simulink model "PI"  (R2015a)
settings: Solver=ode45  StartTime=0.0  StopTime=300  RelTol=1e-3
libraries: fuzblock x1
settings Model: Creator=Q  LastModifiedBy=Q

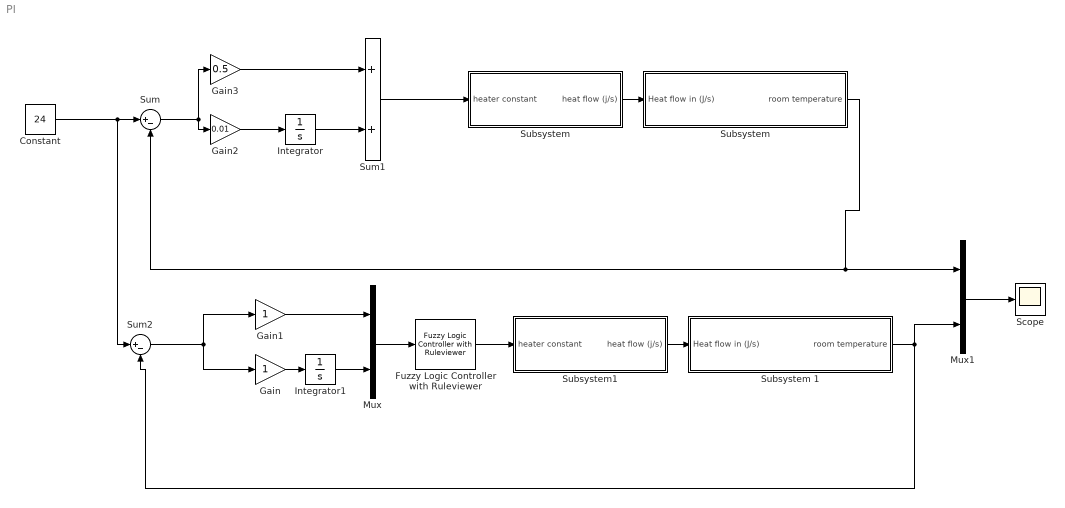
== system PI ==
  Constant : Constant  Value=24
  Fuzzy Logic Controller with Ruleviewer : fuzblock/Fuzzy Logic  Controller  with Ruleviewer  fismatrix=room_heater1  Ts=2
  Gain : Gain
  Gain1 : Gain
  Gain2 : Gain  Gain=0.01
  Gain3 : Gain  Gain=0.5
  Integrator : Integrator  LimitOutput=on  UpperSaturationLimit=1  LowerSaturationLimit=0
  Integrator1 : Integrator  LimitOutput=on  UpperSaturationLimit=1  LowerSaturationLimit=0
  Mux : Mux  Inputs=2
  Mux1 : Mux  Inputs=2
  Scope : Scope
      settings: TimeRange=50  YMin=23.99  YMax=24.15
  Subsystem : Subsystem
  "Subsystem " : Subsystem
  Subsystem 1 : Subsystem
  Subsystem1 : Subsystem
  Sum : Sum  Inputs=|+-
  Sum1 : Sum
  Sum2 : Sum  Inputs=|+-
  wires:
  Subsystem/1(heat flow (j/s)) -> "Subsystem "/1(Heat flow in (J/s))
  "Subsystem "/1(room temperature) -> Sum/2, Mux1/1
  Mux/1 -> Fuzzy Logic Controller with Ruleviewer/1
  Integrator1/1 -> Mux/2
  Gain1/1 -> Mux/1
  Integrator/1 -> Sum1/2
  Gain3/1 -> Sum1/1
  Subsystem1/1(heat flow (j/s)) -> Subsystem 1/1(Heat flow in (J/s))
  Constant/1 -> Sum2/1, Sum/1
  Subsystem 1/1(room temperature) -> Mux1/2, Sum2/2
  Sum2/1 -> Gain/1, Gain1/1
  Fuzzy Logic Controller with Ruleviewer/1 -> Subsystem1/1("heater constant ")
  Mux1/1 -> Scope/1
  Gain/1 -> Integrator1/1
  Sum/1 -> Gain3/1, Gain2/1
  Sum1/1 -> Subsystem/1("heater constant ")
  Gain2/1 -> Integrator/1

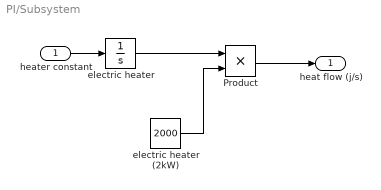
== system PI/Subsystem ==
  "heater constant " : Inport
  Product : Product
  "electric heater " : Integrator  LimitOutput=on  UpperSaturationLimit=1  LowerSaturationLimit=0
  electric heater (2kW) : Constant  Value=2000
  heat flow (j/s) : Outport
  wires:
  "heater constant "/1 -> "electric heater "/1
  "electric heater "/1 -> Product/1
  electric heater (2kW)/1 -> Product/2
  Product/1 -> heat flow (j/s)/1

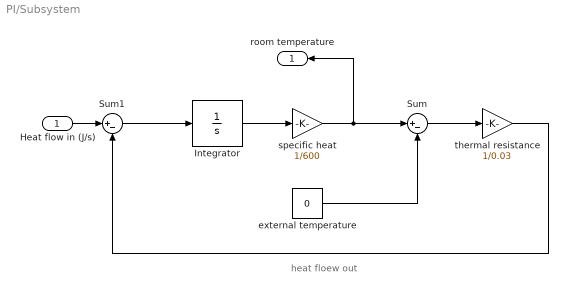
== system PI/Subsystem  ==
  note: heat floew out
  Heat flow in (J/s) : Inport
  Integrator : Integrator
  Sum : Sum  Inputs=|+-
  Sum1 : Sum  Inputs=|+-
  "external temperature  " : Constant  Value=0
  "specific heat " : Gain  Gain=1/600
  thermal resistance : Gain  Gain=1/0.03
  room temperature : Outport
  wires:
  Sum1/1 -> Integrator/1
  Heat flow in (J/s)/1 -> Sum1/1
  Sum/1 -> thermal resistance/1
  Integrator/1 -> "specific heat "/1
  "external temperature  "/1 -> Sum/2
  "specific heat "/1 -> room temperature/1, Sum/1
  thermal resistance/1 -> Sum1/2

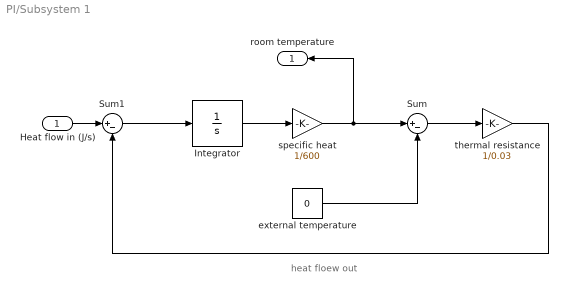
== system PI/Subsystem 1 ==
  note: heat floew out
  Heat flow in (J/s) : Inport
  Integrator : Integrator
  Sum : Sum  Inputs=|+-
  Sum1 : Sum  Inputs=|+-
  "external temperature  " : Constant  Value=0
  "specific heat " : Gain  Gain=1/600
  thermal resistance : Gain  Gain=1/0.03
  room temperature : Outport
  wires:
  Sum1/1 -> Integrator/1
  Heat flow in (J/s)/1 -> Sum1/1
  Sum/1 -> thermal resistance/1
  Integrator/1 -> "specific heat "/1
  "external temperature  "/1 -> Sum/2
  "specific heat "/1 -> room temperature/1, Sum/1
  thermal resistance/1 -> Sum1/2

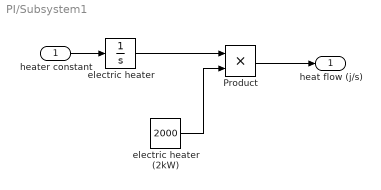
== system PI/Subsystem1 ==
  "heater constant " : Inport
  Product : Product
  "electric heater " : Integrator  LimitOutput=on  UpperSaturationLimit=1  LowerSaturationLimit=0
  electric heater (2kW) : Constant  Value=2000
  heat flow (j/s) : Outport
  wires:
  "heater constant "/1 -> "electric heater "/1
  "electric heater "/1 -> Product/1
  electric heater (2kW)/1 -> Product/2
  Product/1 -> heat flow (j/s)/1
